simulink model "Torque_controller_PBC_standalone_clase_ej_ver2020b"  (R2020b)
settings: Solver=ode5  StartTime=0.0  StopTime=tsim  FixedStep=tstep  MaxStep=1e-4  RelTol=1e-3
PreLoadFcn:
  | % Estructura para parametros del motor de induccion
  | 
  | tsim = 20;
  | tstep = 1e-4;
  | 
  | nomvals = struct('Pnom',745.7,'v_Srmsnom',230,'i_Srmsnom',0,'psi_Rmagnom',0,'w_Rnom',180.64,'tau_Rnom',0);
  | elecparams = struct('n_p',2,'R_S',2.516,'R_R',1.941,'L_S',0.234,'L_R',0.2303,'M',0.2226,'sigma',0,'gamma',0);
  | mechparams = struct('J',0.0062764,'b',0.00011);
  | 
  | nomvals.i_Srmsnom = nomvals.Pnom/nomvals.v_Srmsnom;
  | nomvals.psi_Rmagnom = elecparams.M*nomvals.i_Srmsnom/sqrt(2);
  | nomvals.tau_Rnom = nomvals.Pnom/nomvals.w_Rnom;
  | 
  | elecparams.sigma = elecparams.L_S-(elecparams.M^2/elecparams.L_R);
  | elecparams.gamma = (elecparams.R_S*elecparams.L_R^2+elecparams.R_R*elecparams.M^2)/(elecparams.sigma*elecparams.L_R^2);
  | 
  | MI_params = struct('nomvals',nomvals,'elecparams',elecparams,'mechparams',mechparams);
  | 
  | MI_bus_info = Simulink.Bus.createObject(MI_params);
  | MI_bus = evalin('base', MI_bus_info.busName);
  | 
  | 
  | % Estructura de datos para los parametros del controlador
  | 
  | MI_Contr = struct('psi_Rmagref',MI_params.nomvals.psi_Rmagnom,'epsilon_KiS',1);
  | 
  | MI_Contr_bus = Simulink.Bus.createObject(MI_Contr);
  | 
  | 
  | % Estructura de datos para los perfiles de torque de referencia tau_Rref y torque de carga tau_L
  | % nota: por defecto: tau_Rref == tau_L
  | 
  | % nombre = nombre;
  | % obj.sel_perfil = sel_perfil;
  | 
  | % if obj.sel_perfil ~= 1 && obj.sel_perfil ~= 7
  | %     perfiles.valor_referencia = valor_referencia;
  | % else
  | %     perfiles.valor_referencia = 0;
  | % end
  | 
  | perfiles.sel_perfil = 5;
  | perfiles.valor_referencia = MI_params.nomvals.tau_Rnom/2;
  | 
  | % 1 = constante 0, 2 = 2 escalones, 3 = rampa, 4 = senoidal, 5 = polinomio 7mo orden
  | % 6 = escalones sucesivos hasta torque nominal (% de torque nominal)
  | % 7 = funcion personalizada (timeseries)
  | % 8 = trayectoria 15 segmentos
  | 
  | % 1. Constante 0
  | % 2. Parametros Escalon
  | perfiles.escalon1.valor_inicial = 0;
  | perfiles.escalon1.amplitud = perfiles.valor_referencia;
  | perfiles.escalon1.tiempo_inicio = 2.5;
  | 
  | perfiles.escalon2.valor_inicial = 0;
  | perfiles.escalon2.amplitud = -perfiles.valor_referencia;
  | perfiles.escalon2.tiempo_inicio = 7.5;
  | 
  | % 3. Parametros Rampa
  | perfiles.rampa.tiempo_inicio = 2.5;
  | perfiles.rampa.tiempo_fin = 7.5;
  | perfiles.rampa.valor_inicial = 0;
  | perfiles.rampa.valor_final = perfiles.valor_referencia;
  | perfiles.rampa.pendiente = (perfiles.rampa.valor_final-perfiles.rampa.valor_inicial)...
  |                           /(perfiles.rampa.tiempo_fin-perfiles.rampa.tiempo_inicio);
  | 
  | % 4. Parametros Senoidal
  | perfiles.senoidal.amplitud = perfiles.valor_referencia;
  | perfiles.senoidal.offset = 0;
  | perfiles.senoidal.frecuencia = 3*pi; %Hz
  | perfiles.senoidal.desfase = pi/2;
  | perfiles.senoidal.tiempo_inicio = 2.5;
  | 
  | % 5. Parametros Polinomio 7mo orden
  | perfiles.polinomio7.tiempo.inicial = 2.5;
  | perfiles.polinomio7.tiempo.final = 7.5;
  | perfiles.polinomio7.pos.inicial = 0;
  | perfiles.polinomio7.pos.final = perfiles.valor_referencia;
  | perfiles.polinomio7.vel.inicial = 0;
  | perfiles.polinomio7.vel.final = 0;
  | perfiles.polinomio7.acel.inicial = 0;
  | perfiles.polinomio7.acel.final = 0;
  | perfiles.polinomio7.jerk.inicial = 0;
  | perfiles.polinomio7.jerk.final = 0;
  | 
  | % 6. tren de escalones sucesivos hasta torque nominal
  | perfiles.escalones.tiempo_entre_escalones = 2.5;
  | perfiles.escalones.amplitud = 0.25*perfiles.valor_referencia; %en terminos de tau_Rnom
  | 
  | % % 7. funcion personalizada (timeseries)
  | % perfiles.ts.time = 0:tstep:tsim;
  | % if obj.sel_perfil == 7
  | %     perfil_archivo = valor_referencia;
  | %     perfiles.ts.data = load(perfiles.valor_referencia);
  | % else
  | %     perfil_archivo = "";
  | %     perfiles.ts.data = zeros(size(perfiles.ts.time));
  | % end
  | 
  | % 8. Parametros trayectoria 15 segmentos
  | perfiles.tr15segs.tiempo.inicial = 2.5;
  | perfiles.tr15segs.pos.inicial = 0;
  | perfiles.tr15segs.pos.final = perfiles.valor_referencia;
  | perfiles.tr15segs.vel_path = 5;
  | perfiles.tr15segs.acel_path = 2.5;
  | perfiles.tr15segs.jerk_path = 10;
  | perfiles.tr15segs.snap_path = 100;
  | 
  | tau_Rref = struct('perfiles',perfiles);
  | tau_L = struct('perfiles',perfiles);
  | 
  | Perfil_bus_info = Simulink.Bus.createObject(tau_L.perfiles);
  | Perfil_bus = evalin('base', Perfil_bus_info.busName);
libraries: simulink x4
settings Model: Creator=ferda  LastModifiedBy=HP
settings DebuggingCC: UnconnectedInputMsg=none  UnconnectedOutputMsg=none  UnconnectedLineMsg=none
settings ModelReferenceCC: EnableRefExpFcnMdlSchedulingChecks=off

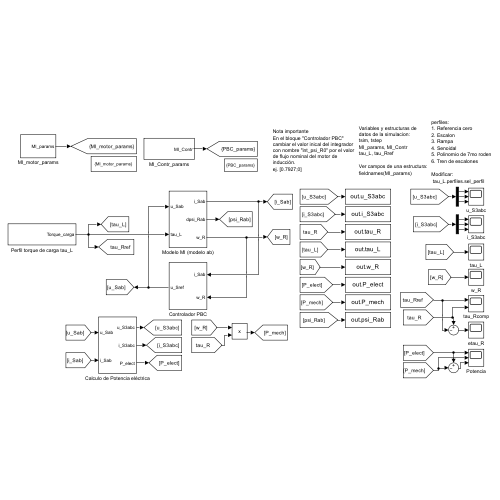
[thumbnail: Simulink's stored preview of the top-level diagram]
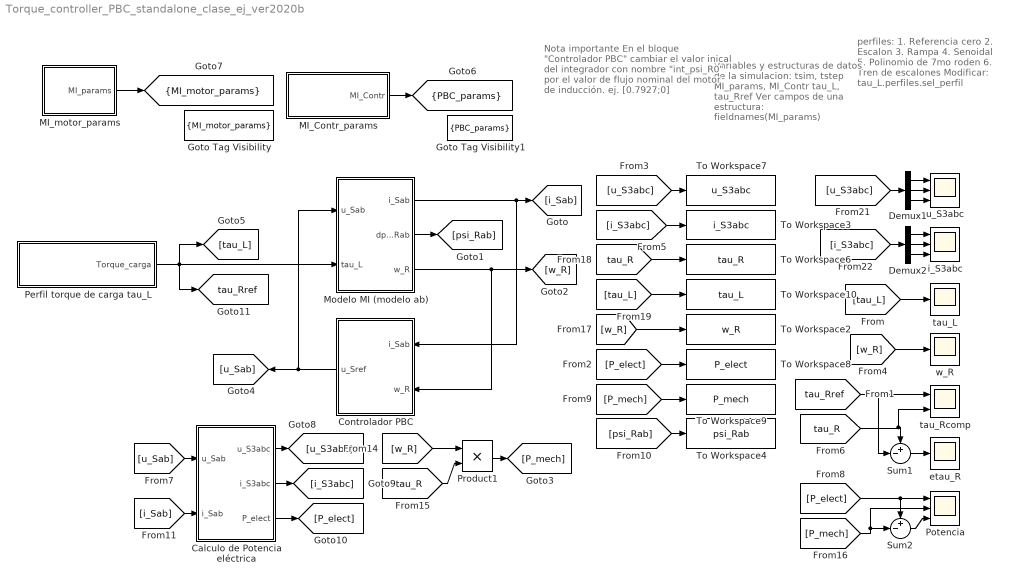
== system Torque_controller_PBC_standalone_clase_ej_ver2020b ==
  note: perfiles:
      | 1. Referencia cero
      | 2. Escalon
      | 3. Rampa
      | 4. Senoidal
      | 5. Polinomio de 7mo roden
      | 6. Tren de escalones
      |
      | Modificar:
      | tau_L.perfiles.sel_perfil
  note: Variables y estructuras de datos de la simulacion:
      | tsim, tstep
      | MI_params, MI_Contr
      | tau_L, tau_Rref
      |
      | Ver campos de una estructura:
      | fieldnames(MI_params)
  note: Nota importante
      | En el bloque "Controlador PBC"
      | cambiar el valor inical del integrador con nombre "int_psi_R0" por el valor de flujo nominal del motor de inducción.
      | ej. [0.7927;0]
  Calculo de Potencia eléctrica : Subsystem
  Controlador PBC : Subsystem
  Demux1 : Demux  Outputs=3
  Demux2 : Demux  Outputs=3
  Goto Tag Visibility : GotoTagVisibility  GotoTag=MI_motor_params
  Goto Tag Visibility1 : GotoTagVisibility  GotoTag=PBC_params
  MI_Contr_params : Subsystem
  MI_motor_params : Subsystem
  Modelo MI (modelo ab) : Subsystem
  Perfil torque de carga tau_L : Subsystem
  Potencia : Scope  NumInputPorts=3
  Product1 : Product
  Sum1 : Sum  Inputs=+-|
  Sum2 : Sum  Inputs=+-|
  To Workspace10 : ToWorkspace  VariableName=tau_L  SaveFormat=Timeseries  SampleTime=-1
  To Workspace2 : ToWorkspace  VariableName=w_R  SaveFormat=Timeseries  SampleTime=-1
  To Workspace3 : ToWorkspace  VariableName=i_S3abc  SaveFormat=Timeseries  SampleTime=-1
  To Workspace4 : ToWorkspace  VariableName=psi_Rab  SaveFormat=Timeseries  SampleTime=-1
  To Workspace6 : ToWorkspace  VariableName=tau_R  SaveFormat=Timeseries  SampleTime=-1
  To Workspace7 : ToWorkspace  VariableName=u_S3abc  SaveFormat=Timeseries  SampleTime=-1
  To Workspace8 : ToWorkspace  VariableName=P_elect  SaveFormat=Timeseries  SampleTime=-1
  To Workspace9 : ToWorkspace  VariableName=P_mech  SaveFormat=Timeseries  SampleTime=-1
  etau_R : Scope
  i_S3abc : Scope  NumInputPorts=3
  tau_L : Scope
  tau_Rcomp : Scope  NumInputPorts=2
  u_S3abc : Scope  NumInputPorts=3
  w_R : Scope
  tag scope: MI_motor_params=scoped, PBC_params=scoped, tau_Rref=global
  wires:
  Controlador PBC/1(u_Sref) -> Modelo MI (modelo ab)/1(u_Sab), [u_Sab]
  Modelo MI (modelo ab)/1(i_Sab) -> Controlador PBC/1(i_Sab), [i_Sab]
  Modelo MI (modelo ab)/2(dpsi_Rab) -> [psi_Rab]
  [tau_Rref] -> Sum1/2, tau_Rcomp/1
  Modelo MI (modelo ab)/3(w_R) -> Controlador PBC/2(w_R), [w_R]
  [w_R] -> w_R/1
  Perfil torque de carga tau_L/1(Torque_carga) -> [tau_Rref], Modelo MI (modelo ab)/2(tau_L), [tau_L]
  [tau_R] -> Sum1/1, tau_Rcomp/2
  Sum2/1 -> Potencia/3
  [i_S3abc] -> Demux2/1
  [u_S3abc] -> Demux1/1
  [P_mech] -> Potencia/2, Sum2/2
  Demux2/1 -> i_S3abc/1
  [P_elect] -> Potencia/1, Sum2/1
  Demux2/3 -> i_S3abc/3
  Demux2/2 -> i_S3abc/2
  Demux1/2 -> u_S3abc/2
  [u_Sab] -> Calculo de Potencia eléctrica/1(u_Sab)
  Calculo de Potencia eléctrica/3(P_elect) -> [P_elect]
  Calculo de Potencia eléctrica/2(i_S3abc) -> [i_S3abc]
  Demux1/3 -> u_S3abc/3
  [i_Sab] -> Calculo de Potencia eléctrica/2(i_Sab)
  Calculo de Potencia eléctrica/1(u_S3abc) -> [u_S3abc]
  Demux1/1 -> u_S3abc/1
  [P_elect] -> To Workspace8/1
  [w_R] -> To Workspace2/1
  [u_S3abc] -> To Workspace7/1
  [P_mech] -> To Workspace9/1
  [tau_R] -> To Workspace6/1
  [i_S3abc] -> To Workspace3/1
  [tau_L] -> To Workspace10/1
  [psi_Rab] -> To Workspace4/1
  [tau_R] -> Product1/2
  Product1/1 -> [P_mech]
  [w_R] -> Product1/1
  MI_Contr_params/1(MI_Contr) -> [PBC_params]
  [tau_L] -> tau_L/1
  MI_motor_params/1(MI_params) -> [MI_motor_params]
  Sum1/1 -> etau_R/1

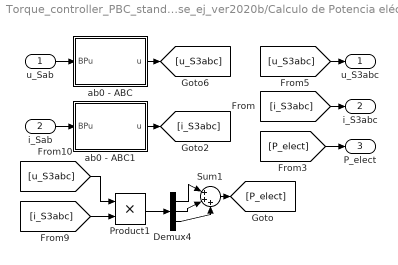
== system Torque_controller_PBC_standalone_clase_ej_ver2020b/Calculo de Potencia eléctrica ==
  u_Sab : Inport
  i_Sab : Inport  Port=2
  Demux4 : Demux  Outputs=3
  Product1 : Product
  Sum1 : Sum  Inputs=|+++
  ab0 - ABC : MATLAB Function  TreatAsAtomicUnit=on
  ab0 - ABC1 : MATLAB Function  TreatAsAtomicUnit=on
  u_S3abc : Outport
  i_S3abc : Outport  Port=2
  P_elect : Outport  Port=3
  wires:
  Demux4/1 -> Sum1/1
  [i_S3abc] -> Product1/2
  i_Sab/1 -> ab0 - ABC1/1(BPu)
  Demux4/3 -> Sum1/3
  [u_S3abc] -> Product1/1
  Demux4/2 -> Sum1/2
  Product1/1 -> Demux4/1
  u_Sab/1 -> ab0 - ABC/1(BPu)
  [u_S3abc] -> u_S3abc/1
  [i_S3abc] -> i_S3abc/1
  ab0 - ABC/1(u) -> [u_S3abc]
  ab0 - ABC1/1(u) -> [i_S3abc]
  Sum1/1 -> [P_elect]
  [P_elect] -> P_elect/1

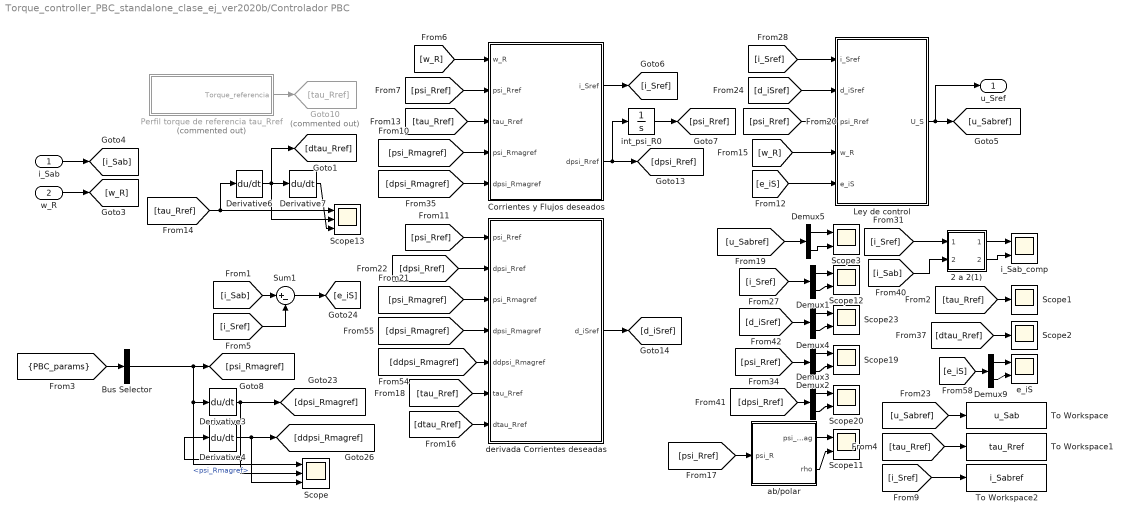
== system Torque_controller_PBC_standalone_clase_ej_ver2020b/Controlador PBC ==
  i_Sab : Inport
  w_R : Inport  Port=2
  2 a 2(1) : Subsystem
  Bus Selector : BusSelector  OutputSignals=psi_Rmagref
  Corrientes y Flujos deseados : Subsystem
  Demux{1..5,9} (6 alike) : Demux  Outputs=2
  Derivative{3..4,6..7} (4 alike) : Derivative
  Goto10 : Goto  Commented=on  GotoTag=tau_Rref
  Ley de control : Subsystem
  Perfil torque de referencia tau_Rref : Subsystem  Commented=on
  Scope : Scope  NumInputPorts=3
  Scope1 : Scope
  Scope{3,11..12,19..20,23} (6 alike) : Scope  NumInputPorts=2
  Scope13 : Scope  NumInputPorts=3
  Scope2 : Scope
  Sum1 : Sum  Inputs=|+-
  To Workspace : ToWorkspace  VariableName=u_Sab  SaveFormat=Timeseries  SampleTime=-1
  To Workspace1 : ToWorkspace  VariableName=tau_Rref  SaveFormat=Timeseries  SampleTime=-1
  To Workspace2 : ToWorkspace  VariableName=i_Sabref  SaveFormat=Timeseries  SampleTime=-1
  ab/polar : MATLAB Function  TreatAsAtomicUnit=on
  derivada Corrientes deseadas : Subsystem
  e_iS : Scope  NumInputPorts=2
  i_Sab_comp : Scope  NumInputPorts=2
  int_psi_R0 : Integrator  InitialCondition=[0.510324559349035;0]
  u_Sref : Outport
  wires:
  Derivative3/1 -> Scope/2, Derivative4/1, [dpsi_Rmagref]
  Derivative4/1 -> [ddpsi_Rmagref], Scope/3
  Bus Selector/1 -> Derivative3/1, Scope/1, [psi_Rmagref]  "<psi_Rmagref>"
  i_Sab/1 -> [i_Sab]
  [tau_Rref] -> Corrientes y Flujos deseados/3(tau_Rref)
  [w_R] -> Corrientes y Flujos deseados/1(w_R)
  int_psi_R0/1 -> [psi_Rref]
  Corrientes y Flujos deseados/2(dpsi_Rref) -> int_psi_R0/1, [dpsi_Rref]
  [psi_Rref] -> Corrientes y Flujos deseados/2(psi_Rref)
  [psi_Rmagref] -> Corrientes y Flujos deseados/4(psi_Rmagref)
  [dpsi_Rmagref] -> Corrientes y Flujos deseados/5(dpsi_Rmagref)
  [psi_Rref] -> derivada Corrientes deseadas/1(psi_Rref)
  [dpsi_Rref] -> derivada Corrientes deseadas/2(dpsi_Rref)
  [psi_Rmagref] -> derivada Corrientes deseadas/3(psi_Rmagref)
  [dpsi_Rmagref] -> derivada Corrientes deseadas/4(dpsi_Rmagref)
  [ddpsi_Rmagref] -> derivada Corrientes deseadas/5(ddpsi_Rmagref)
  [tau_Rref] -> derivada Corrientes deseadas/6(tau_Rref)
  [dtau_Rref] -> derivada Corrientes deseadas/7(dtau_Rref)
  derivada Corrientes deseadas/1(d_iSref) -> [d_iSref]
  [e_iS] -> Demux9/1
  Demux9/1 -> e_iS/1
  Demux9/2 -> e_iS/2
  [i_Sab] -> Sum1/1
  [i_Sref] -> Sum1/2
  Sum1/1 -> [e_iS]
  [i_Sref] -> Ley de control/1(i_Sref)
  [d_iSref] -> Ley de control/2(d_iSref)
  [psi_Rref] -> Ley de control/3(psi_Rref)
  [w_R] -> Ley de control/4(w_R)
  Ley de control/1(U_S) -> u_Sref/1, [u_Sabref]
  [e_iS] -> Ley de control/5(e_iS)
  Derivative7/1 -> Scope13/3
  Derivative6/1 -> [dtau_Rref], Derivative7/1, Scope13/2
  2 a 2(1)/2(Out2) -> i_Sab_comp/2
  2 a 2(1)/1(Out1) -> i_Sab_comp/1
  [i_Sab] -> 2 a 2(1)/2(In2)
  [i_Sref] -> 2 a 2(1)/1(In1)
  w_R/1 -> [w_R]
  [tau_Rref] -> Scope1/1
  [PBC_params] -> Bus Selector/1
  Corrientes y Flujos deseados/1(i_Sref) -> [i_Sref]
  [u_Sabref] -> To Workspace/1
  [tau_Rref] -> To Workspace1/1
  [i_Sref] -> To Workspace2/1
  ab/polar/1(psi_Rmag) -> Scope11/1
  [psi_Rref] -> ab/polar/1(psi_R)
  Demux4/1 -> Scope23/1
  [i_Sref] -> Demux1/1
  Demux2/2 -> Scope19/2
  [psi_Rref] -> Demux2/1
  Demux3/2 -> Scope20/2
  Demux3/1 -> Scope20/1
  [d_iSref] -> Demux4/1
  Demux4/2 -> Scope23/2
  Demux2/1 -> Scope19/1
  [dpsi_Rref] -> Demux3/1
  Demux1/2 -> Scope12/2
  Demux1/1 -> Scope12/1
  [dtau_Rref] -> Scope2/1
  [tau_Rref] -> Derivative6/1, Scope13/1
  Perfil torque de referencia tau_Rref/1(Torque_referencia) -> Goto10/1
  Demux5/1 -> Scope3/1
  Demux5/2 -> Scope3/2
  [u_Sabref] -> Demux5/1
  ab/polar/2(rho) -> Scope11/2

== system Torque_controller_PBC_standalone_clase_ej_ver2020b/MI_Contr_params ==
  Bus Creator : BusCreator  Inputs=2
  Display : Display
  Display1 : Display
  MATLAB Function : MATLAB Function  TreatAsAtomicUnit=on
  MI_Contr : Outport
  wires:
  MATLAB Function/1(psi_Rmagref) -> Display/1, Bus Creator/1
  MATLAB Function/2(epsilon_KiS) -> Display1/1, Bus Creator/2
  [MI_motor_params] -> MATLAB Function/1(MI_motor_params)
  Bus Creator/1 -> MI_Contr/1

== system Torque_controller_PBC_standalone_clase_ej_ver2020b/MI_motor_params ==
  MI_motor_params : MATLAB Function  TreatAsAtomicUnit=on
  MI_params : Outport
  wires:
  MI_motor_params/1(MI_params) -> MI_params/1

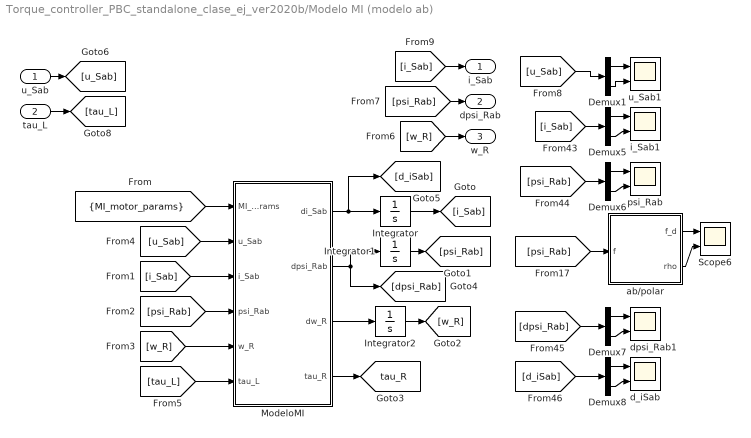
== system Torque_controller_PBC_standalone_clase_ej_ver2020b/Modelo MI (modelo ab) ==
  u_Sab : Inport
  tau_L : Inport  Port=2
  Demux{1,5..8} (5 alike) : Demux  Outputs=2
  Integrator : Integrator
  Integrator1 : Integrator
  Integrator2 : Integrator
  ModeloMI : MATLAB Function  TreatAsAtomicUnit=on
  Scope6 : Scope  NumInputPorts=2
  ab/polar : MATLAB Function  TreatAsAtomicUnit=on
  d_iSab : Scope  NumInputPorts=2
  dpsi_Rab1 : Scope  NumInputPorts=2
  i_Sab1 : Scope  NumInputPorts=2
  psi_Rab : Scope  NumInputPorts=2
  u_Sab1 : Scope  NumInputPorts=2
  i_Sab : Outport
  dpsi_Rab : Outport  Port=2
  w_R : Outport  Port=3
  tag scope: tau_R=global
  wires:
  ModeloMI/1(di_Sab) -> Integrator/1, [d_iSab]
  ModeloMI/2(dpsi_Rab) -> [dpsi_Rab], Integrator1/1
  [w_R] -> ModeloMI/5(w_R)
  [psi_Rab] -> ModeloMI/4(psi_Rab)
  Integrator2/1 -> [w_R]
  [i_Sab] -> ModeloMI/3(i_Sab)
  ModeloMI/3(dw_R) -> Integrator2/1
  Integrator1/1 -> [psi_Rab]
  u_Sab/1 -> [u_Sab]
  ModeloMI/4(tau_R) -> [tau_R]
  Demux7/1 -> dpsi_Rab1/1
  Demux7/2 -> dpsi_Rab1/2
  [d_iSab] -> Demux8/1
  Demux8/2 -> d_iSab/2
  Demux8/1 -> d_iSab/1
  [dpsi_Rab] -> Demux7/1
  Integrator/1 -> [i_Sab]
  [MI_motor_params] -> ModeloMI/1(MI_motor_params)
  Demux6/2 -> psi_Rab/2
  Demux5/1 -> i_Sab1/1
  [psi_Rab] -> Demux6/1
  Demux5/2 -> i_Sab1/2
  Demux6/1 -> psi_Rab/1
  [i_Sab] -> Demux5/1
  ab/polar/2(rho) -> Scope6/2
  ab/polar/1(f_d) -> Scope6/1
  [psi_Rab] -> ab/polar/1(f)
  [u_Sab] -> ModeloMI/2(u_Sab)
  tau_L/1 -> [tau_L]
  [tau_L] -> ModeloMI/6(tau_L)
  [i_Sab] -> i_Sab/1
  [psi_Rab] -> dpsi_Rab/1
  [w_R] -> w_R/1
  [u_Sab] -> Demux1/1
  Demux1/1 -> u_Sab1/1
  Demux1/2 -> u_Sab1/2

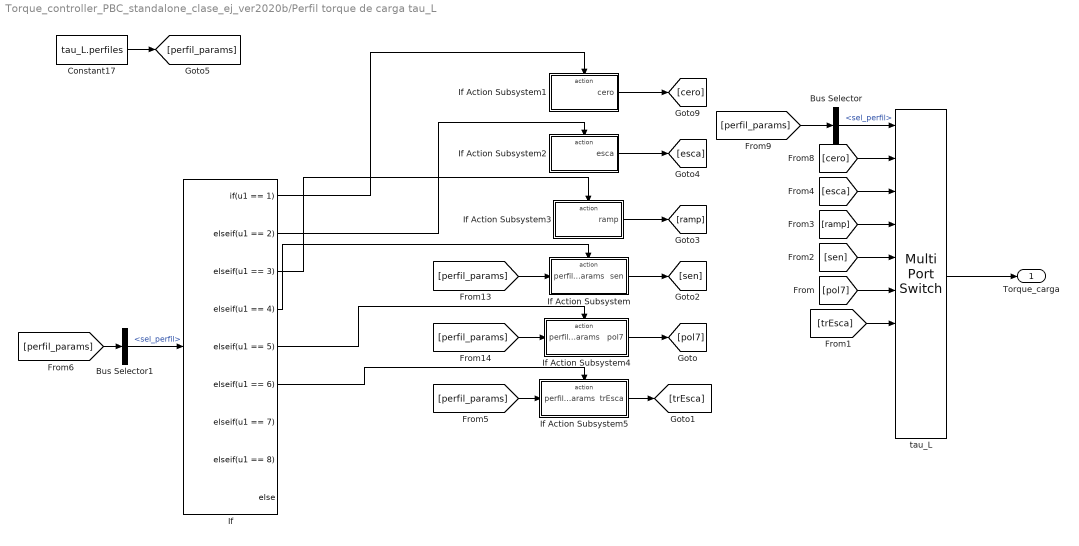
== system Torque_controller_PBC_standalone_clase_ej_ver2020b/Perfil torque de carga tau_L ==
  Bus Selector : BusSelector  OutputSignals=sel_perfil
  Bus Selector1 : BusSelector  OutputSignals=sel_perfil
  Constant17 : Constant  Value=tau_L.perfiles  OutDataTypeStr=Bus: Perfil_bus
  If : If  IfExpression=u1 == 1  ElseIfExpressions=u1 == 2,u1 == 3,u1 == 4,u1 == 5,u1 == 6,u1 == 7,u1 == 8
  If Action Subsystem : Subsystem  TreatAsAtomicUnit=on
  If Action Subsystem1 : Subsystem  TreatAsAtomicUnit=on
  If Action Subsystem2 : Subsystem  TreatAsAtomicUnit=on
  If Action Subsystem3 : Subsystem  TreatAsAtomicUnit=on
  If Action Subsystem4 : Subsystem  TreatAsAtomicUnit=on
  If Action Subsystem5 : Subsystem  TreatAsAtomicUnit=on
  tau_L : MultiPortSwitch  Inputs=9
  Torque_carga : Outport
  wires:
  tau_L/1 -> Torque_carga/1
  [ramp] -> tau_L/4
  [trEsca] -> tau_L/7
  [pol7] -> tau_L/6
  [sen] -> tau_L/5
  [esca] -> tau_L/3
  Bus Selector/1 -> tau_L/1  "<sel_perfil>"
  [perfil_params] -> Bus Selector/1
  If Action Subsystem/1(sen) -> [sen]
  [perfil_params] -> Bus Selector1/1
  Bus Selector1/1 -> If/1  "<sel_perfil>"
  If/4 -> If Action Subsystem/Action
  If Action Subsystem1/1(cero) -> [cero]
  [cero] -> tau_L/2
  [perfil_params] -> If Action Subsystem/1(perfil_params)
  If/1 -> If Action Subsystem1/Action
  If Action Subsystem2/1(esca) -> [esca]
  If/2 -> If Action Subsystem2/Action
  If Action Subsystem3/1(ramp) -> [ramp]
  If/3 -> If Action Subsystem3/Action
  [perfil_params] -> If Action Subsystem4/1(perfil_params)
  If/5 -> If Action Subsystem4/Action
  If Action Subsystem4/1(pol7) -> [pol7]
  If Action Subsystem5/1(trEsca) -> [trEsca]
  [perfil_params] -> If Action Subsystem5/1(perfil_params)
  If/6 -> If Action Subsystem5/Action
  Constant17/1 -> [perfil_params]

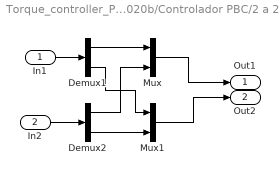
== system Torque_controller_PBC_standalone_clase_ej_ver2020b/Controlador PBC/2 a 2(1) ==
  In1 : Inport
  In2 : Inport  Port=2
  Demux1 : Demux  Outputs=2
  Demux2 : Demux  Outputs=2
  Mux : Mux  Inputs=2
  Mux1 : Mux  Inputs=2
  Out1 : Outport
  Out2 : Outport  Port=2
  wires:
  Demux2/1 -> Mux/2
  Mux/1 -> Out1/1
  In2/1 -> Demux2/1
  In1/1 -> Demux1/1
  Demux1/1 -> Mux/1
  Demux1/2 -> Mux1/1
  Mux1/1 -> Out2/1
  Demux2/2 -> Mux1/2

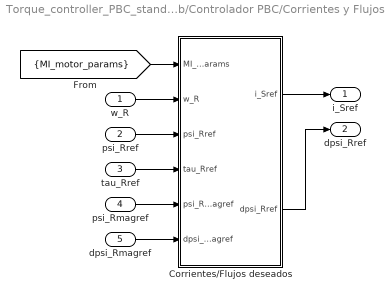
== system Torque_controller_PBC_standalone_clase_ej_ver2020b/Controlador PBC/Corrientes y Flujos deseados ==
  w_R : Inport
  psi_Rref : Inport  Port=2
  tau_Rref : Inport  Port=3
  psi_Rmagref : Inport  Port=4
  dpsi_Rmagref : Inport  Port=5
  Corrientes/Flujos deseados : MATLAB Function  TreatAsAtomicUnit=on
  i_Sref : Outport
  dpsi_Rref : Outport  Port=2
  wires:
  tau_Rref/1 -> Corrientes/Flujos deseados/4(tau_Rref)
  Corrientes/Flujos deseados/1(i_Sref) -> i_Sref/1
  psi_Rref/1 -> Corrientes/Flujos deseados/3(psi_Rref)
  w_R/1 -> Corrientes/Flujos deseados/2(w_R)
  Corrientes/Flujos deseados/2(dpsi_Rref) -> dpsi_Rref/1
  psi_Rmagref/1 -> Corrientes/Flujos deseados/5(psi_Rmagref)
  dpsi_Rmagref/1 -> Corrientes/Flujos deseados/6(dpsi_Rmagref)
  [MI_motor_params] -> Corrientes/Flujos deseados/1(MI_motor_params)

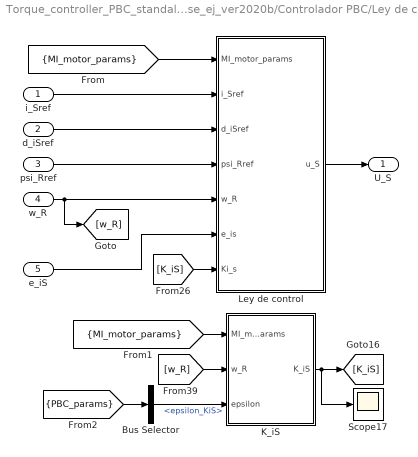
== system Torque_controller_PBC_standalone_clase_ej_ver2020b/Controlador PBC/Ley de control ==
  i_Sref : Inport
  d_iSref : Inport  Port=2
  psi_Rref : Inport  Port=3
  w_R : Inport  Port=4
  e_iS : Inport  Port=5
  Bus Selector : BusSelector  OutputSignals=epsilon_KiS
  K_iS : MATLAB Function  TreatAsAtomicUnit=on
  Ley de control : MATLAB Function  TreatAsAtomicUnit=on
  Scope17 : Scope
  U_S : Outport
  wires:
  [K_iS] -> Ley de control/7(Ki_s)
  d_iSref/1 -> Ley de control/3(d_iSref)
  psi_Rref/1 -> Ley de control/4(psi_Rref)
  i_Sref/1 -> Ley de control/2(i_Sref)
  Ley de control/1(u_S) -> U_S/1
  w_R/1 -> [w_R], Ley de control/5(w_R)
  e_iS/1 -> Ley de control/6(e_is)
  Bus Selector/1 -> K_iS/3(epsilon)  "<epsilon_KiS>"
  K_iS/1(K_iS) -> Scope17/1, [K_iS]
  [w_R] -> K_iS/2(w_R)
  [MI_motor_params] -> Ley de control/1(MI_motor_params)
  [MI_motor_params] -> K_iS/1(MI_motor_params)
  [PBC_params] -> Bus Selector/1

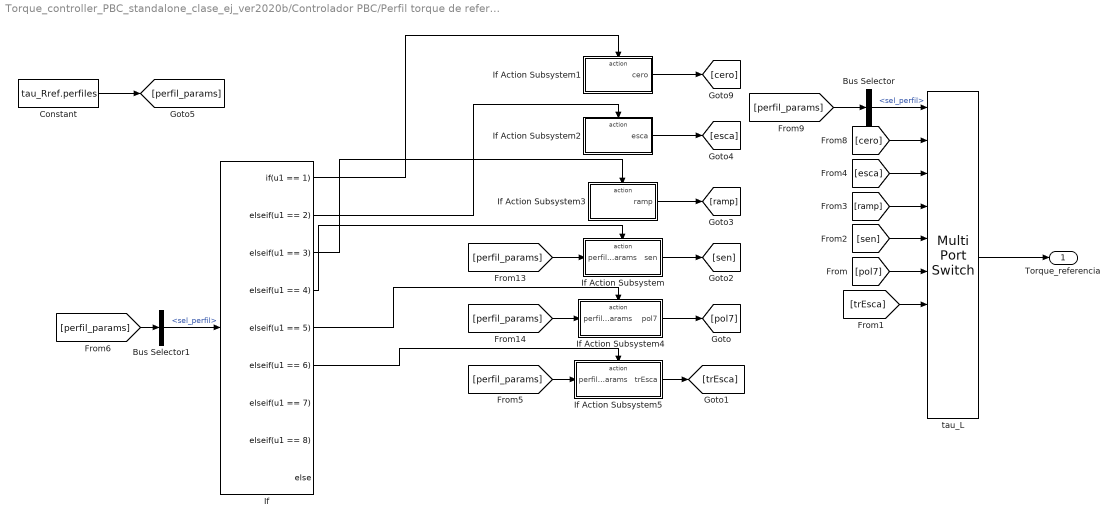
== system Torque_controller_PBC_standalone_clase_ej_ver2020b/Controlador PBC/Perfil torque de referencia tau_Rref ==
  Bus Selector : BusSelector  OutputSignals=sel_perfil
  Bus Selector1 : BusSelector  OutputSignals=sel_perfil
  Constant : Constant  Value=tau_Rref.perfiles  OutDataTypeStr=Bus: Perfil_bus
  If : If  IfExpression=u1 == 1  ElseIfExpressions=u1 == 2,u1 == 3,u1 == 4,u1 == 5,u1 == 6,u1 == 7,u1 == 8
  If Action Subsystem : Subsystem  TreatAsAtomicUnit=on
  If Action Subsystem1 : Subsystem  TreatAsAtomicUnit=on
  If Action Subsystem2 : Subsystem  TreatAsAtomicUnit=on
  If Action Subsystem3 : Subsystem  TreatAsAtomicUnit=on
  If Action Subsystem4 : Subsystem  TreatAsAtomicUnit=on
  If Action Subsystem5 : Subsystem  TreatAsAtomicUnit=on
  tau_L : MultiPortSwitch  Inputs=9
  Torque_referencia : Outport
  wires:
  tau_L/1 -> Torque_referencia/1
  [ramp] -> tau_L/4
  [trEsca] -> tau_L/7
  [pol7] -> tau_L/6
  [sen] -> tau_L/5
  [esca] -> tau_L/3
  Bus Selector/1 -> tau_L/1  "<sel_perfil>"
  [perfil_params] -> Bus Selector/1
  If Action Subsystem/1(sen) -> [sen]
  [perfil_params] -> Bus Selector1/1
  Bus Selector1/1 -> If/1  "<sel_perfil>"
  If/4 -> If Action Subsystem/Action
  If Action Subsystem1/1(cero) -> [cero]
  [cero] -> tau_L/2
  [perfil_params] -> If Action Subsystem/1(perfil_params)
  If/1 -> If Action Subsystem1/Action
  If Action Subsystem2/1(esca) -> [esca]
  If/2 -> If Action Subsystem2/Action
  If Action Subsystem3/1(ramp) -> [ramp]
  If/3 -> If Action Subsystem3/Action
  [perfil_params] -> If Action Subsystem4/1(perfil_params)
  If/5 -> If Action Subsystem4/Action
  If Action Subsystem4/1(pol7) -> [pol7]
  If Action Subsystem5/1(trEsca) -> [trEsca]
  [perfil_params] -> If Action Subsystem5/1(perfil_params)
  If/6 -> If Action Subsystem5/Action
  Constant/1 -> [perfil_params]

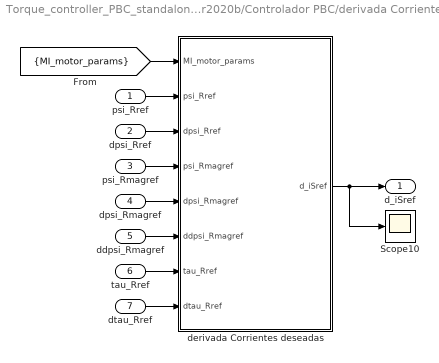
== system Torque_controller_PBC_standalone_clase_ej_ver2020b/Controlador PBC/derivada Corrientes deseadas ==
  psi_Rref : Inport
  dpsi_Rref : Inport  Port=2
  psi_Rmagref : Inport  Port=3
  dpsi_Rmagref : Inport  Port=4
  ddpsi_Rmagref : Inport  Port=5
  tau_Rref : Inport  Port=6
  dtau_Rref : Inport  Port=7
  Scope10 : Scope
  derivada Corrientes deseadas : MATLAB Function  TreatAsAtomicUnit=on
  d_iSref : Outport
  wires:
  dpsi_Rref/1 -> derivada Corrientes deseadas/3(dpsi_Rref)
  tau_Rref/1 -> derivada Corrientes deseadas/7(tau_Rref)
  dtau_Rref/1 -> derivada Corrientes deseadas/8(dtau_Rref)
  dpsi_Rmagref/1 -> derivada Corrientes deseadas/5(dpsi_Rmagref)
  derivada Corrientes deseadas/1(d_iSref) -> Scope10/1, d_iSref/1
  psi_Rmagref/1 -> derivada Corrientes deseadas/4(psi_Rmagref)
  psi_Rref/1 -> derivada Corrientes deseadas/2(psi_Rref)
  ddpsi_Rmagref/1 -> derivada Corrientes deseadas/6(ddpsi_Rmagref)
  [MI_motor_params] -> derivada Corrientes deseadas/1(MI_motor_params)

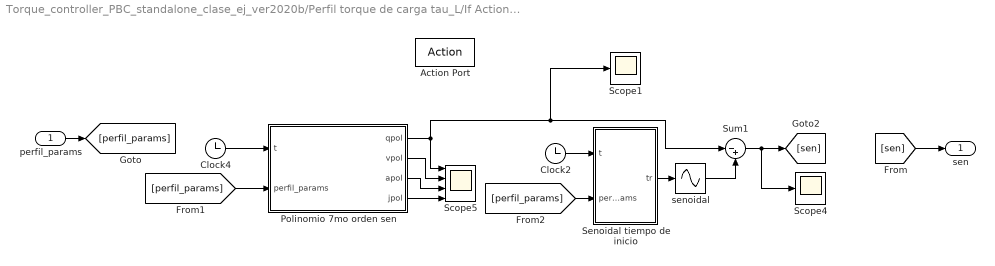
== system Torque_controller_PBC_standalone_clase_ej_ver2020b/Perfil torque de carga tau_L/If Action Subsystem ==
  perfil_params : Inport
  Action Port : ActionPort  ActionPortLabel=elseif(u1 == 4)
  Clock2 : Clock
  Clock4 : Clock
  Polinomio 7mo orden sen : MATLAB Function  TreatAsAtomicUnit=on
  Scope1 : Scope
  Scope4 : Scope
  Scope5 : Scope  NumInputPorts=4
  Senoidal tiempo de inicio : MATLAB Function  TreatAsAtomicUnit=on
  Sum1 : Sum  Inputs=|-+
  senoidal : Sin  TimeSource=Use external signal  Frequency=6.2832  Phase=1.5708  SampleTime=0
  sen : Outport
  wires:
  Clock4/1 -> Polinomio 7mo orden sen/1(t)
  Polinomio 7mo orden sen/1(qpol) -> Scope1/1, Sum1/1, Scope5/1
  Sum1/1 -> Scope4/1, [sen]
  Polinomio 7mo orden sen/4(jpol) -> Scope5/4
  Polinomio 7mo orden sen/3(apol) -> Scope5/3
  Clock2/1 -> Senoidal tiempo de inicio/1(t)
  [perfil_params] -> Polinomio 7mo orden sen/2(perfil_params)
  Polinomio 7mo orden sen/2(vpol) -> Scope5/2
  senoidal/1 -> Sum1/2
  Senoidal tiempo de inicio/1(tr) -> senoidal/1
  [sen] -> sen/1
  perfil_params/1 -> [perfil_params]
  [perfil_params] -> Senoidal tiempo de inicio/2(perfil_params)

== system Torque_controller_PBC_standalone_clase_ej_ver2020b/Perfil torque de carga tau_L/If Action Subsystem1 ==
  Action Port : ActionPort  ActionPortLabel=if(u1 == 1)
  Constant : Constant  Value=0
  cero : Outport
  wires:
  Constant/1 -> cero/1

== system Torque_controller_PBC_standalone_clase_ej_ver2020b/Perfil torque de carga tau_L/If Action Subsystem2 ==
  Action Port : ActionPort  ActionPortLabel=elseif(u1 == 2)
  Scope3 : Scope
  Sum : Sum  Inputs=|++
  escalon1 : Step  Time=2.5  After=0.70582  SampleTime=0
  escalon2 : Step  Time=7.5  After=-0.70582  SampleTime=0
  esca : Outport
  wires:
  escalon2/1 -> Sum/2
  escalon1/1 -> Sum/1
  Sum/1 -> [esca], Scope3/1
  [esca] -> esca/1

== system Torque_controller_PBC_standalone_clase_ej_ver2020b/Perfil torque de carga tau_L/If Action Subsystem3 ==
  Action Port : ActionPort  ActionPortLabel=elseif(u1 == 3)
  Scope2 : Scope
  Sum2 : Sum  Inputs=|++
  rampa1 : simulink/Sources/Ramp  slope=0.02064  start=2.5  InitialOutput=0
  rampa2 : simulink/Sources/Ramp  slope=-0.02064  start=7.5  InitialOutput=0
  ramp : Outport
  wires:
  rampa2/1 -> Sum2/2
  rampa1/1 -> Sum2/1
  Sum2/1 -> Scope2/1, [ramp]
  [ramp] -> ramp/1

== system Torque_controller_PBC_standalone_clase_ej_ver2020b/Perfil torque de carga tau_L/If Action Subsystem4 ==
  perfil_params : Inport
  Action Port : ActionPort  ActionPortLabel=elseif(u1 == 5)
  Clock1 : Clock
  Polinomio 7mo orden tau_L : MATLAB Function  TreatAsAtomicUnit=on
  Scope : Scope  NumInputPorts=4
  pol7 : Outport
  wires:
  Polinomio 7mo orden tau_L/4(jpol) -> Scope/4
  Polinomio 7mo orden tau_L/1(qpol) -> Scope/1, [pol7]
  Polinomio 7mo orden tau_L/2(vpol) -> Scope/2
  Clock1/1 -> Polinomio 7mo orden tau_L/1(t)
  Polinomio 7mo orden tau_L/3(apol) -> Scope/3
  perfil_params/1 -> Polinomio 7mo orden tau_L/2(perfil_params)
  [pol7] -> pol7/1

== system Torque_controller_PBC_standalone_clase_ej_ver2020b/Perfil torque de carga tau_L/If Action Subsystem5 ==
  perfil_params : Inport
  Action Port : ActionPort  ActionPortLabel=elseif(u1 == 6)
  Clock : Clock
  Scope1 : Scope
  Tren de esca : MATLAB Function  TreatAsAtomicUnit=on
  trEsca : Outport
  wires:
  Tren de esca/1(q) -> Scope1/1, [trEsca]
  Clock/1 -> Tren de esca/1(t)
  perfil_params/1 -> Tren de esca/2(perfil_params)
  [trEsca] -> trEsca/1

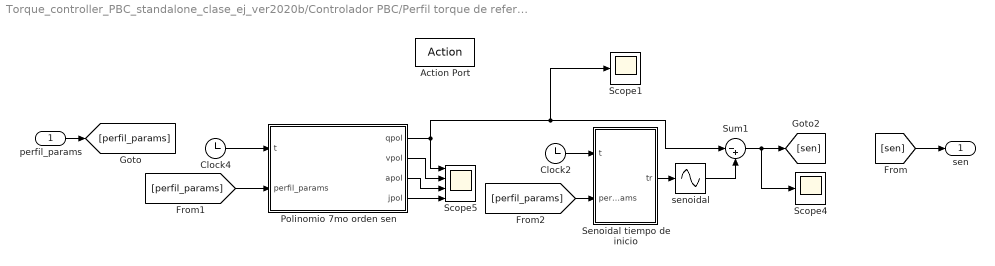
== system Torque_controller_PBC_standalone_clase_ej_ver2020b/Controlador PBC/Perfil torque de referencia tau_Rref/If Action Subsystem ==
  perfil_params : Inport
  Action Port : ActionPort  ActionPortLabel=elseif(u1 == 4)
  Clock2 : Clock
  Clock4 : Clock
  Polinomio 7mo orden sen : MATLAB Function  TreatAsAtomicUnit=on
  Scope1 : Scope
  Scope4 : Scope
  Scope5 : Scope  NumInputPorts=4
  Senoidal tiempo de inicio : MATLAB Function  TreatAsAtomicUnit=on
  Sum1 : Sum  Inputs=|-+
  senoidal : Sin  TimeSource=Use external signal  Frequency=6.2832  Phase=1.5708  SampleTime=0
  sen : Outport
  wires:
  Clock4/1 -> Polinomio 7mo orden sen/1(t)
  Polinomio 7mo orden sen/1(qpol) -> Scope1/1, Sum1/1, Scope5/1
  Sum1/1 -> Scope4/1, [sen]
  Polinomio 7mo orden sen/4(jpol) -> Scope5/4
  Polinomio 7mo orden sen/3(apol) -> Scope5/3
  Clock2/1 -> Senoidal tiempo de inicio/1(t)
  [perfil_params] -> Polinomio 7mo orden sen/2(perfil_params)
  Polinomio 7mo orden sen/2(vpol) -> Scope5/2
  senoidal/1 -> Sum1/2
  Senoidal tiempo de inicio/1(tr) -> senoidal/1
  [sen] -> sen/1
  perfil_params/1 -> [perfil_params]
  [perfil_params] -> Senoidal tiempo de inicio/2(perfil_params)

== system Torque_controller_PBC_standalone_clase_ej_ver2020b/Controlador PBC/Perfil torque de referencia tau_Rref/If Action Subsystem1 ==
  Action Port : ActionPort  ActionPortLabel=if(u1 == 1)
  Constant : Constant  Value=0
  cero : Outport
  wires:
  Constant/1 -> cero/1

== system Torque_controller_PBC_standalone_clase_ej_ver2020b/Controlador PBC/Perfil torque de referencia tau_Rref/If Action Subsystem2 ==
  Action Port : ActionPort  ActionPortLabel=elseif(u1 == 2)
  Scope3 : Scope
  Sum : Sum  Inputs=|++
  escalon1 : Step  Time=2.5  After=0.70582  SampleTime=0
  escalon2 : Step  Time=7.5  After=-0.70582  SampleTime=0
  esca : Outport
  wires:
  escalon2/1 -> Sum/2
  escalon1/1 -> Sum/1
  Sum/1 -> [esca], Scope3/1
  [esca] -> esca/1

== system Torque_controller_PBC_standalone_clase_ej_ver2020b/Controlador PBC/Perfil torque de referencia tau_Rref/If Action Subsystem3 ==
  Action Port : ActionPort  ActionPortLabel=elseif(u1 == 3)
  Scope2 : Scope
  Sum2 : Sum  Inputs=|++
  rampa1 : simulink/Sources/Ramp  slope=0.02064  start=2.5  InitialOutput=0
  rampa2 : simulink/Sources/Ramp  slope=-0.02064  start=7.5  InitialOutput=0
  ramp : Outport
  wires:
  rampa2/1 -> Sum2/2
  rampa1/1 -> Sum2/1
  Sum2/1 -> Scope2/1, [ramp]
  [ramp] -> ramp/1

== system Torque_controller_PBC_standalone_clase_ej_ver2020b/Controlador PBC/Perfil torque de referencia tau_Rref/If Action Subsystem4 ==
  perfil_params : Inport
  Action Port : ActionPort  ActionPortLabel=elseif(u1 == 5)
  Clock1 : Clock
  Polinomio 7mo orden tau_L : MATLAB Function  TreatAsAtomicUnit=on
  Scope : Scope  NumInputPorts=4
  pol7 : Outport
  wires:
  Polinomio 7mo orden tau_L/4(jpol) -> Scope/4
  Polinomio 7mo orden tau_L/1(qpol) -> Scope/1, [pol7]
  Polinomio 7mo orden tau_L/2(vpol) -> Scope/2
  Clock1/1 -> Polinomio 7mo orden tau_L/1(t)
  Polinomio 7mo orden tau_L/3(apol) -> Scope/3
  perfil_params/1 -> Polinomio 7mo orden tau_L/2(perfil_params)
  [pol7] -> pol7/1

== system Torque_controller_PBC_standalone_clase_ej_ver2020b/Controlador PBC/Perfil torque de referencia tau_Rref/If Action Subsystem5 ==
  perfil_params : Inport
  Action Port : ActionPort  ActionPortLabel=elseif(u1 == 6)
  Clock : Clock
  Scope1 : Scope
  Tren de esca : MATLAB Function  TreatAsAtomicUnit=on
  trEsca : Outport
  wires:
  Tren de esca/1(q) -> Scope1/1, [trEsca]
  Clock/1 -> Tren de esca/1(t)
  perfil_params/1 -> Tren de esca/2(perfil_params)
  [trEsca] -> trEsca/1

== matlab function Torque_controller_PBC_standalone_clase_ej_ver2020b/Perfil torque de carga tau_L/If Action Subsystem/Polinomio 7mo orden sen ==
  data: t input; perfil_params input; qpol output; vpol output; apol output; jpol output
function [qpol,vpol,apol,jpol] = fcn(t,perfil_params)

%Trayectoria de referencia

q0 = 0;
q1 = perfil_params.senoidal.amplitud;

% v0 = perfil_params.polinomio7.vel.inicial;
% v1 = perfil_params.polinomio7.vel.final;
% 
% ac0 = perfil_params.polinomio7.acel.inicial;
% ac1 = perfil_params.polinomio7.acel.final;
% 
% j0 = perfil_params.polinomio7.jerk.inicial;
% j1 = perfil_params.polinomio7.jerk.inicial;

if perfil_params.senoidal.tiempo_inicio-1>0
    t0 = perfil_params.senoidal.tiempo_inicio-1;
else
    t0 = 0;
end
t1 = perfil_params.senoidal.tiempo_inicio;

% Coeficientes de un polinomio de 7mo grado
[qpol,vpol,apol,jpol] = pol7(t,q1,q0,t0,t1);

function [qpol,vpol,apol,jpol] = pol7(t,q0,q1,t0,t1)
%Trayectoria de referencia

% q0 = 0;
% q1 = 1;

v0 = 0;
v1 = 0;

ac0 = 0;
ac1 = 0;

j0 = 0;
j1 = 0;

% t0 = t1;
% t1 = ;

% Coeficientes de un polinomio de 7mo grado

h = q1 - q0;
T = t1 - t0;

a = zeros(7+1,1);

a(1) = q0;
a(2) = v0;
a(3) = ac0/2;
a(4) = j0/6;
a(5) = (210*h-T*((30*ac0-15*ac1)*T+(4*j0+j1)*T^2+120*v0+90*v1))/(6*T^4);
a(6) = (-168*h-T*((20*ac0-14*ac1)*T+(2*j0+j1)*T^2+90*v0+78*v1))/(2*T^5);
a(7) = (420*h-T*((45*ac0-39*ac1)*T+(4*j0+3*j1)*T^2+216*v0+204*v1))/(6*T^6);
a(8) = (-120*h-T*((12*ac0-12*ac1)*T+(j0+j1)*T^2+60*v0+60*v1))/(6*T^7);

qa = flip(a')';
va = polyder(qa')';
aa = polyder(va')';
ja = polyder(aa')';


t_interval = (t-t0).*double(t>=t0).*double(t<t1) + (t1-t0).*double(t>=t1);

qpol = polyval(qa,t_interval);
vpol = polyval(va,t_interval);
apol = polyval(aa,t_interval);
jpol = polyval(ja,t_interval);

== matlab function Torque_controller_PBC_standalone_clase_ej_ver2020b/MI_Contr_params/MATLAB Function ==
  data: psi_Rmagref output; MI_motor_params input Bus: MI_bus; epsilon_KiS output
function [psi_Rmagref,epsilon_KiS] = fcn(MI_motor_params)

psi_Rmagref = MI_motor_params.nomvals.psi_Rmagnom;
epsilon_KiS = 1;

== matlab function Torque_controller_PBC_standalone_clase_ej_ver2020b/Perfil torque de carga tau_L/If Action Subsystem4/Polinomio 7mo orden tau_L ==
  data: t input; perfil_params input; qpol output; vpol output; apol output; jpol output
function [qpol,vpol,apol,jpol] = fcn(t,perfil_params)

%Trayectoria de referencia

q0 = perfil_params.polinomio7.pos.inicial;
q1 = perfil_params.polinomio7.pos.final;

% v0 = perfil_params.polinomio7.vel.inicial;
% v1 = perfil_params.polinomio7.vel.final;
% 
% ac0 = perfil_params.polinomio7.acel.inicial;
% ac1 = perfil_params.polinomio7.acel.final;
% 
% j0 = perfil_params.polinomio7.jerk.inicial;
% j1 = perfil_params.polinomio7.jerk.inicial;

t0 = perfil_params.polinomio7.tiempo.inicial;
t1 = perfil_params.polinomio7.tiempo.final;

% Coeficientes de un polinomio de 7mo grado
[qpol,vpol,apol,jpol] = pol7(t,q0,q1,t0,t1);

function [qpol,vpol,apol,jpol] = pol7(t,q0,q1,t0,t1)
%Trayectoria de referencia

% q0 = 0;
% q1 = 1;

v0 = 0;
v1 = 0;

ac0 = 0;
ac1 = 0;

j0 = 0;
j1 = 0;

% t0 = t1;
% t1 = ;

% Coeficientes de un polinomio de 7mo grado

h = q1 - q0;
T = t1 - t0;

a = zeros(7+1,1);

a(1) = q0;
a(2) = v0;
a(3) = ac0/2;
a(4) = j0/6;
a(5) = (210*h-T*((30*ac0-15*ac1)*T+(4*j0+j1)*T^2+120*v0+90*v1))/(6*T^4);
a(6) = (-168*h-T*((20*ac0-14*ac1)*T+(2*j0+j1)*T^2+90*v0+78*v1))/(2*T^5);
a(7) = (420*h-T*((45*ac0-39*ac1)*T+(4*j0+3*j1)*T^2+216*v0+204*v1))/(6*T^6);
a(8) = (-120*h-T*((12*ac0-12*ac1)*T+(j0+j1)*T^2+60*v0+60*v1))/(6*T^7);

qa = flip(a')';
va = polyder(qa')';
aa = polyder(va')';
ja = polyder(aa')';


t_interval = (t-t0).*double(t>=t0).*double(t<t1) + (t1-t0).*double(t>=t1);

qpol = polyval(qa,t_interval);
vpol = polyval(va,t_interval);
apol = polyval(aa,t_interval);
jpol = polyval(ja,t_interval);

== matlab function Torque_controller_PBC_standalone_clase_ej_ver2020b/Perfil torque de carga tau_L/If Action Subsystem/Senoidal tiempo de inicio ==
  data: t input; tr output; perfil_params input
function tr = fcn(t,perfil_params)

t1 = perfil_params.senoidal.tiempo_inicio;

if t < t1
    tr = 0;
else
    tr = t - t1;
end

== matlab function Torque_controller_PBC_standalone_clase_ej_ver2020b/Perfil torque de carga tau_L/If Action Subsystem5/Tren de esca ==
  data: t input; q output; perfil_params input
function q = fcn(t,perfil_params)

q = trEsca(t,perfil_params);


function q = trEsca(t,perfil_params)
referencia = perfil_params.valor_referencia;
amplitud = perfil_params.escalones.amplitud;
tstep = perfil_params.escalones.tiempo_entre_escalones;


num_escalones = ceil(referencia/amplitud);

if floor(t/tstep)<num_escalones
    q = amplitud*floor(t/tstep);
else
    q = amplitud*num_escalones;
end

== matlab function Torque_controller_PBC_standalone_clase_ej_ver2020b/Calculo de Potencia eléctrica/ab0 - ABC ==
  data: BPu input size=[2,1]; u output size=[3,1]
function u = fcn(BPu)

BPu = vertcat(BPu,0);

% Power invariant
BP = Clarke_transform(1);

u = BP^-1*BPu;



function BP = Clarke_transform(opt_power_invariant)
if opt_power_invariant == 0
    BP = 2/3*[1,-1/2,-1/2;
              0,sqrt(3)/2,-sqrt(3)/2;
              1/2,1/2,1/2];
else
    % Power invariant
    BP = sqrt(2/3)*[1,-1/2,-1/2;
                    0,sqrt(3)/2,-sqrt(3)/2;
                    1/sqrt(2),1/sqrt(2),1/sqrt(2)];
end

== matlab function Torque_controller_PBC_standalone_clase_ej_ver2020b/Calculo de Potencia eléctrica/ab0 - ABC1 ==
  data: BPu input size=[2,1]; u output size=[3,1]
function u = fcn(BPu)

BPu = vertcat(BPu,0);

% Power invariant
BP = Clarke_transform(1);

u = BP^-1*BPu;

function BP = Clarke_transform(opt_power_invariant)
if opt_power_invariant == 0
    BP = 2/3*[1,-1/2,-1/2;
              0,sqrt(3)/2,-sqrt(3)/2;
              1/2,1/2,1/2];
else
    % Power invariant
    BP = sqrt(2/3)*[1,-1/2,-1/2;
                    0,sqrt(3)/2,-sqrt(3)/2;
                    1/sqrt(2),1/sqrt(2),1/sqrt(2)];
end

== matlab function Torque_controller_PBC_standalone_clase_ej_ver2020b/Controlador PBC/ab//polar ==
  data: psi_R input; psi_Rmag output; rho output
function [psi_Rmag,rho] = fcn(psi_R)

[psi_Rmag,rho] = Polar_transform(psi_R);

function [mag,angle] = Polar_transform(u)
u1 = u(1);
u2 = u(2);

mag = sqrt(u1^2+u2^2);
angle = atan2(u2,u1);

== matlab function Torque_controller_PBC_standalone_clase_ej_ver2020b/Controlador PBC/Perfil torque de referencia tau_Rref/If Action Subsystem/Polinomio 7mo orden sen ==
  data: t input; perfil_params input; qpol output; vpol output; apol output; jpol output
function [qpol,vpol,apol,jpol] = fcn(t,perfil_params)

%Trayectoria de referencia

q0 = 0;
q1 = perfil_params.senoidal.amplitud;

% v0 = perfil_params.polinomio7.vel.inicial;
% v1 = perfil_params.polinomio7.vel.final;
% 
% ac0 = perfil_params.polinomio7.acel.inicial;
% ac1 = perfil_params.polinomio7.acel.final;
% 
% j0 = perfil_params.polinomio7.jerk.inicial;
% j1 = perfil_params.polinomio7.jerk.inicial;

if perfil_params.senoidal.tiempo_inicio-1>0
    t0 = perfil_params.senoidal.tiempo_inicio-1;
else
    t0 = 0;
end
t1 = perfil_params.senoidal.tiempo_inicio;

% Coeficientes de un polinomio de 7mo grado
[qpol,vpol,apol,jpol] = pol7(t,q1,q0,t0,t1);

function [qpol,vpol,apol,jpol] = pol7(t,q0,q1,t0,t1)
%Trayectoria de referencia

% q0 = 0;
% q1 = 1;

v0 = 0;
v1 = 0;

ac0 = 0;
ac1 = 0;

j0 = 0;
j1 = 0;

% t0 = t1;
% t1 = ;

% Coeficientes de un polinomio de 7mo grado

h = q1 - q0;
T = t1 - t0;

a = zeros(7+1,1);

a(1) = q0;
a(2) = v0;
a(3) = ac0/2;
a(4) = j0/6;
a(5) = (210*h-T*((30*ac0-15*ac1)*T+(4*j0+j1)*T^2+120*v0+90*v1))/(6*T^4);
a(6) = (-168*h-T*((20*ac0-14*ac1)*T+(2*j0+j1)*T^2+90*v0+78*v1))/(2*T^5);
a(7) = (420*h-T*((45*ac0-39*ac1)*T+(4*j0+3*j1)*T^2+216*v0+204*v1))/(6*T^6);
a(8) = (-120*h-T*((12*ac0-12*ac1)*T+(j0+j1)*T^2+60*v0+60*v1))/(6*T^7);

qa = flip(a')';
va = polyder(qa')';
aa = polyder(va')';
ja = polyder(aa')';


t_interval = (t-t0).*double(t>=t0).*double(t<t1) + (t1-t0).*double(t>=t1);

qpol = polyval(qa,t_interval);
vpol = polyval(va,t_interval);
apol = polyval(aa,t_interval);
jpol = polyval(ja,t_interval);

== matlab function Torque_controller_PBC_standalone_clase_ej_ver2020b/Controlador PBC/Perfil torque de referencia tau_Rref/If Action Subsystem/Senoidal tiempo de inicio ==
  data: t input; tr output; perfil_params input
function tr = fcn(t,perfil_params)

t1 = perfil_params.senoidal.tiempo_inicio;

if t < t1
    tr = 0;
else
    tr = t - t1;
end

== matlab function Torque_controller_PBC_standalone_clase_ej_ver2020b/Controlador PBC/Perfil torque de referencia tau_Rref/If Action Subsystem4/Polinomio 7mo orden tau_L ==
  data: t input; perfil_params input; qpol output; vpol output; apol output; jpol output
function [qpol,vpol,apol,jpol] = fcn(t,perfil_params)

%Trayectoria de referencia

q0 = perfil_params.polinomio7.pos.inicial;
q1 = perfil_params.polinomio7.pos.final;

% v0 = perfil_params.polinomio7.vel.inicial;
% v1 = perfil_params.polinomio7.vel.final;
% 
% ac0 = perfil_params.polinomio7.acel.inicial;
% ac1 = perfil_params.polinomio7.acel.final;
% 
% j0 = perfil_params.polinomio7.jerk.inicial;
% j1 = perfil_params.polinomio7.jerk.inicial;

t0 = perfil_params.polinomio7.tiempo.inicial;
t1 = perfil_params.polinomio7.tiempo.final;

% Coeficientes de un polinomio de 7mo grado
[qpol,vpol,apol,jpol] = pol7(t,q0,q1,t0,t1);


function [qpol,vpol,apol,jpol] = pol7(t,q0,q1,t0,t1)
%Trayectoria de referencia

% q0 = 0;
% q1 = 1;

v0 = 0;
v1 = 0;

ac0 = 0;
ac1 = 0;

j0 = 0;
j1 = 0;

% t0 = t1;
% t1 = ;

% Coeficientes de un polinomio de 7mo grado

h = q1 - q0;
T = t1 - t0;

a = zeros(7+1,1);

a(1) = q0;
a(2) = v0;
a(3) = ac0/2;
a(4) = j0/6;
a(5) = (210*h-T*((30*ac0-15*ac1)*T+(4*j0+j1)*T^2+120*v0+90*v1))/(6*T^4);
a(6) = (-168*h-T*((20*ac0-14*ac1)*T+(2*j0+j1)*T^2+90*v0+78*v1))/(2*T^5);
a(7) = (420*h-T*((45*ac0-39*ac1)*T+(4*j0+3*j1)*T^2+216*v0+204*v1))/(6*T^6);
a(8) = (-120*h-T*((12*ac0-12*ac1)*T+(j0+j1)*T^2+60*v0+60*v1))/(6*T^7);

qa = flip(a')';
va = polyder(qa')';
aa = polyder(va')';
ja = polyder(aa')';


t_interval = (t-t0).*double(t>=t0).*double(t<t1) + (t1-t0).*double(t>=t1);

qpol = polyval(qa,t_interval);
vpol = polyval(va,t_interval);
apol = polyval(aa,t_interval);
jpol = polyval(ja,t_interval);

== matlab function Torque_controller_PBC_standalone_clase_ej_ver2020b/Controlador PBC/Perfil torque de referencia tau_Rref/If Action Subsystem5/Tren de esca ==
  data: t input; q output; perfil_params input
function q = fcn(t,perfil_params)

q = trEsca(t,perfil_params);

function q = trEsca(t,perfil_params)
referencia = perfil_params.valor_referencia;
amplitud = perfil_params.escalones.amplitud;
tstep = perfil_params.escalones.tiempo_entre_escalones;


num_escalones = ceil(referencia/amplitud);

if floor(t/tstep)<num_escalones
    q = amplitud*floor(t/tstep);
else
    q = amplitud*num_escalones;
end

== matlab function Torque_controller_PBC_standalone_clase_ej_ver2020b/Controlador PBC/Corrientes y Flujos deseados/Corrientes//Flujos deseados ==
  data: MI_motor_params input Bus: MI_bus; w_R input; i_Sref output size=[2 1]; psi_Rref input size=[2,1]; tau_Rref input; psi_Rmagref input; dpsi_Rmagref input; dpsi_Rref output size=[2,1]
function [i_Sref,dpsi_Rref] = fcn(MI_motor_params,w_R,psi_Rref,tau_Rref,psi_Rmagref,dpsi_Rmagref)


% i_Sref = PBC_Torque_Controller.i_Sref(MI_motor_params,psi_Rref,tau_Rref,psi_Rmagref,dpsi_Rmagref);
% dpsi_Rref = PBC_Torque_Controller.dpsi_Ref(MI_motor_params,w_R,psi_Rref,tau_Rref,psi_Rmagref,dpsi_Rmagref);

R_S = MI_motor_params.elecparams.R_R;
R_R = MI_motor_params.elecparams.R_R;
L_S = MI_motor_params.elecparams.L_S;
L_R = MI_motor_params.elecparams.L_R;
M = MI_motor_params.elecparams.M;
n_p = MI_motor_params.elecparams.n_p;
J = MI_motor_params.elecparams.J;
b = MI_motor_params.elecparams.b;

sigma = MI_motor_params.elecparams.sigma;
gamma = MI_motor_params.elecparams.gamma;


psi_Raref = psi_Rref(1);
psi_Rbref = psi_Rref(2);

psi_Raref = psi_Rref(1);
psi_Rbref = psi_Rref(2);

%% Escribir Ecuaciones del controlador




%% %%%%%%%%%%%%%%%%%%%%

i_Sref = [i_Saref;i_Sbref];
dpsi_Rref = [dpsi_Raref;dpsi_Rbref];

== matlab function Torque_controller_PBC_standalone_clase_ej_ver2020b/Modelo MI (modelo ab)/ModeloMI ==
  data: MI_motor_params input Bus: MI_bus; di_Sab output double size=[2 1]; dpsi_Rab output double size=[2 1]; dw_R output size=1; u_Sab input double size=[2 1]; i_Sab input double size=[2 1]; psi_Rab input double size=[2 1]; w_R input double size=1; tau_R output size=1; tau_L input
function [di_Sab,dpsi_Rab,dw_R,tau_R] = fcn(MI_motor_params,u_Sab,i_Sab,psi_Rab,w_R,tau_L)

% [di_Sab,dpsi_Rab,dw_R,tau_R] = MI_model.MI_space_state(MI_motor_params,u_Sab,i_Sab,psi_Rab,w_R,tau_L);

%R_S = MI_motor_params.elecparams.R_S;
R_R = MI_motor_params.elecparams.R_R;
%L_S = MI_motor_params.elecparams.L_S;
L_R = MI_motor_params.elecparams.L_R;
M = MI_motor_params.elecparams.M;
n_p = MI_motor_params.elecparams.n_p;

J = MI_motor_params.mechparams.J;
b = MI_motor_params.mechparams.b;

sigma = MI_motor_params.elecparams.sigma;
gamma = MI_motor_params.elecparams.gamma;
% sigma = L_S - M^2/L_R;
% gamma = M^2*R_R/(sigma*L_R^2)+R_S/sigma;


u_Sa = u_Sab(1);
u_Sb = u_Sab(2);

i_Sa = i_Sab(1);
i_Sb = i_Sab(2);

psi_Ra = psi_Rab(1);
psi_Rb = psi_Rab(2);

tau_R = n_p*M/L_R*(i_Sb*psi_Ra-i_Sa*psi_Rb);

x = [i_Sa;i_Sb;psi_Ra;psi_Rb];

A = [-gamma      , 0            , (M*R_R)/(sigma*L_R^2)    , (n_p*M)/(sigma*L_R)*w_R ;
     0           , -gamma       , -(n_p*M)/(sigma*L_R)*w_R , (M*R_R)/(sigma*L_R^2)   ; 
     (R_R*M)/L_R , 0            , -R_R/L_R                 , -n_p*w_R                ;
     0           , (R_R*M)/L_R  , n_p*w_R                  , -R_R/L_R                ];

B = [1/sigma , 0       ;
     0       , 1/sigma ;
     0       , 0       ;
     0       , 0       ];

dx = A*x + B*[u_Sa;u_Sb];

di_Sab = dx(1:2);
dpsi_Rab = dx(3:4);

dw_R = (1/J)*tau_R - (b/J)*w_R - (1/J)*tau_L;

== matlab function Torque_controller_PBC_standalone_clase_ej_ver2020b/Controlador PBC/Ley de control/Ley de control ==
  data: MI_motor_params input Bus: MI_bus; i_Sref input size=[2,1]; d_iSref input size=[2,1]; u_S output size=[2 1]; psi_Rref input size=[2,1]; w_R input; e_is input; Ki_s input
function u_S = fcn(MI_motor_params,i_Sref,d_iSref,psi_Rref,w_R,e_is,Ki_s)

% u_S = PBC_Torque_Controller.ley_control_uS(MI_motor_params,i_Sref,d_iSref,psi_Rref,w_R,e_is,Ki_s);


R_S = MI_motor_params.elecparams.R_R;
R_R = MI_motor_params.elecparams.R_R;
L_S = MI_motor_params.elecparams.L_S;
L_R = MI_motor_params.elecparams.L_R;
M = MI_motor_params.elecparams.M;
n_p = MI_motor_params.elecparams.n_p;
J = MI_motor_params.elecparams.J;
b = MI_motor_params.elecparams.b;

sigma = MI_motor_params.elecparams.sigma;
gamma = MI_motor_params.elecparams.gamma;


di_Saref = d_iSref(1);
di_Sbref = d_iSref(2);

i_Saref = i_Sref(1);
i_Sbref = i_Sref(2);

psi_Raref = psi_Rref(1);
psi_Rbref = psi_Rref(2);

e_iSa = e_is(1);
e_iSb = e_is(2);

%% Escribir Ecuaciones del controlador




%% %%%%%%%%%%%%%%%%%%%%

u_S = [u_Sa;u_Sb];

== matlab function Torque_controller_PBC_standalone_clase_ej_ver2020b/MI_motor_params/MI_motor_params ==
  data: MI_params output Bus: MI_bus
function MI_params = fcn()


% MI 0.4 hp
%300,380,361.283,1,15.6,23.2,1.44,1.5,1.42,0.000711,0.00014

% MI 1hp
%745.7,230,180.64,2,2.516,1.9461,0.234,0.2303,0.2226,0.0062764,0.00011

% MI 5hp
%3728.5,460,183.2595,2,1.115,1.083,0.20967,0.20967,0.2037,0.02,0.005752

nomvals = struct('Pnom',745.7,'v_Srmsnom',230,'i_Srmsnom',0,'psi_Rmagnom',0,'w_Rnom',180.64,'tau_Rnom',0);
elecparams = struct('n_p',2,'R_S',2.516,'R_R',1.941,'L_S',0.234,'L_R',0.2303,'M',0.2226,'sigma',0,'gamma',0);
mechparams = struct('J',0.0062764,'b',0.00011);

nomvals.i_Srmsnom = nomvals.Pnom/nomvals.v_Srmsnom;
nomvals.psi_Rmagnom = elecparams.M*nomvals.i_Srmsnom/sqrt(2);
nomvals.tau_Rnom = nomvals.Pnom/nomvals.w_Rnom;

elecparams.sigma = elecparams.L_S-(elecparams.M^2/elecparams.L_R);
elecparams.gamma = (elecparams.R_S*elecparams.L_R^2+elecparams.R_R*elecparams.M^2)/(elecparams.sigma*elecparams.L_R^2);

MI_params = struct('nomvals',nomvals,'elecparams',elecparams,'mechparams',mechparams);

== matlab function Torque_controller_PBC_standalone_clase_ej_ver2020b/Modelo MI (modelo ab)/ab//polar ==
  data: f input; f_d output; rho output
function [f_d,rho] = fcn(f)

[f_d,rho] = Polar_transform(f);

function [mag,angle] = Polar_transform(u)
u1 = u(1);
u2 = u(2);

mag = sqrt(u1^2+u2^2);
angle = atan2(u2,u1);

== matlab function Torque_controller_PBC_standalone_clase_ej_ver2020b/Controlador PBC/derivada Corrientes deseadas/derivada Corrientes deseadas ==
  data: MI_motor_params input Bus: MI_bus; d_iSref output size=[2 1]; psi_Rref input size=[2,1]; dpsi_Rref input size=[2,1]; psi_Rmagref input; dpsi_Rmagref input; ddpsi_Rmagref input; tau_Rref input; dtau_Rref input
function d_iSref = fcn(MI_motor_params,psi_Rref,dpsi_Rref,psi_Rmagref,dpsi_Rmagref,ddpsi_Rmagref,tau_Rref,dtau_Rref)

% d_iSref = PBC_Torque_Controller.d_iSref(MI_motor_params,psi_Rref,dpsi_Rref,psi_Rmagref,dpsi_Rmagref,ddpsi_Rmagref,tau_Rref,dtau_Rref);

R_S = MI_motor_params.elecparams.R_R;
R_R = MI_motor_params.elecparams.R_R;
L_S = MI_motor_params.elecparams.L_S;
L_R = MI_motor_params.elecparams.L_R;
M = MI_motor_params.elecparams.M;
n_p = MI_motor_params.elecparams.n_p;
J = MI_motor_params.elecparams.J;
b = MI_motor_params.elecparams.b;

sigma = MI_motor_params.elecparams.sigma;
gamma = MI_motor_params.elecparams.gamma;


dpsi_Raref = dpsi_Rref(1);
dpsi_Rbref = dpsi_Rref(2);

psi_Raref = psi_Rref(1);
psi_Rbref = psi_Rref(2);

%% Escribir Ecuaciones del controlador




%% %%%%%%%%%%%%%%%%%%%%


d_iSref = [d_iSaref;d_iSbref];

== matlab function Torque_controller_PBC_standalone_clase_ej_ver2020b/Controlador PBC/Ley de control/K_iS ==
  data: MI_motor_params input Bus: MI_bus; w_R input; epsilon input; K_iS output
function K_iS = fcn(MI_motor_params,w_R,epsilon)

% K_iS = PBC_Torque_Controller.K_iS(MI_motor_params,w_R,epsilon);

R_S = MI_motor_params.elecparams.R_R;
R_R = MI_motor_params.elecparams.R_R;
L_S = MI_motor_params.elecparams.L_S;
L_R = MI_motor_params.elecparams.L_R;
M = MI_motor_params.elecparams.M;
n_p = MI_motor_params.elecparams.n_p;
J = MI_motor_params.elecparams.J;
b = MI_motor_params.elecparams.b;

sigma = MI_motor_params.elecparams.sigma;
gamma = MI_motor_params.elecparams.gamma;


%% Escribir Ecuaciones del controlador




%% %%%%%%%%%%%%%%%%%%%%
